simulink model "simulacion_lab5"  (R2020a)
settings: Solver=VariableStepAuto  StartTime=0.0  StopTime=10.0  RelTol=1e-3
settings Model: Creator=Miguel Gutierrez  LastModifiedBy=Miguel Gutierrez

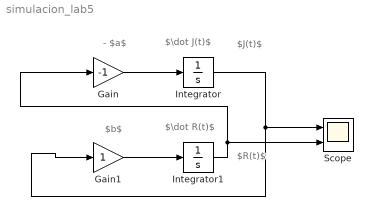
== system simulacion_lab5 ==
  note: - $a$
  note: $\dot J(t)$
  note: $J(t)$
  note: $b$
  note: $\dot R(t)$
  note: $R(t)$
  Gain : Gain  Gain=-1
  Gain1 : Gain
  Integrator : Integrator  InitialCondition=5
  Integrator1 : Integrator
  Scope : Scope  NumInputPorts=2
  wires:
  Gain/1 -> Integrator/1
  Gain1/1 -> Integrator1/1
  Integrator1/1 -> Scope/2, Gain/1
  Integrator/1 -> Gain1/1, Scope/1
